simulink model "polyfitraspi"  (R2022a)
settings: Solver=VariableStepAuto  StartTime=0.0  StopTime=10.0  RelTol=1e-3
libraries: raspberrypiAVlib x2
settings Model: Creator=sanz  LastModifiedBy=sanz

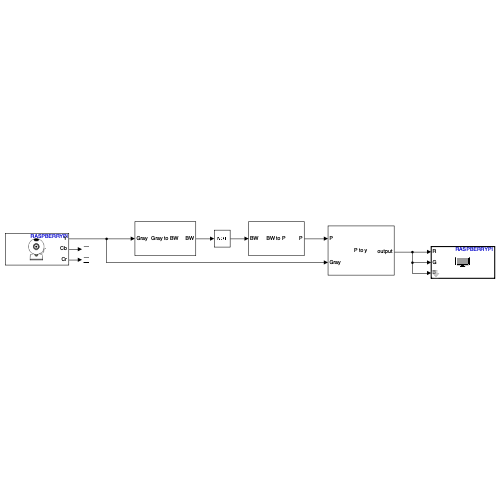
[thumbnail: Simulink's stored preview of the top-level diagram]
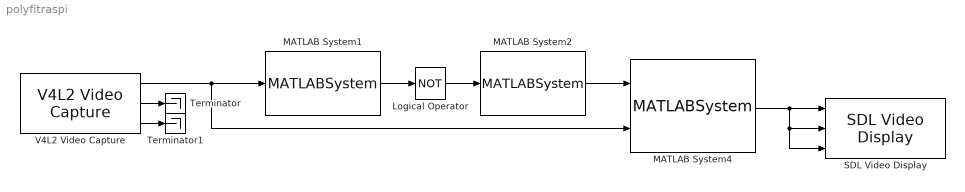
== system polyfitraspi ==
  Logical Operator : Logic  Operator=NOT  AllPortsSameDT=off  OutDataTypeStr=boolean
  MATLAB System1 : MATLABSystem  System=FrameBinarizeSystem  SimulateUsing=Code generation
      mask Type: FrameBinarizeSystem
      mask Display:
      | disp('Gray to BW');
      | port_label('input',1,'Gray');
      | port_label('output',1,'BW');
  MATLAB System2 : MATLABSystem  System=PolyfitSystem  Deg=4  SimulateUsing=Code generation
      mask Type: PolyfitSystem
      mask Display:
      | disp('BW to P');
      | port_label('input',1,'BW');
      | port_label('output',1,'P');
  MATLAB System4 : MATLABSystem  System=PolyvalSystem  SimulateUsing=Code generation
      mask Type: PolyvalSystem
      mask Display:
      | disp('P to y');
      | port_label('input',1,'P');
      | port_label('input',2,'Gray');
      | port_label('output',1,'output');
  SDL Video Display : raspberrypiAVlib/SDL Video Display  title=SDL Video Display  pixelFormat=RGB  pixelOrder=Planar  rowMajor=on  blockPlatform=Raspberry Pi
      settings: SourceProductBaseCode=SC_BEAGLEBONE_BLUE,EMBEDDEDLINUX,NVIDIA,RASPPIIO
  Terminator : Terminator
  Terminator1 : Terminator
  V4L2 Video Capture : raspberrypiAVlib/V4L2 Video Capture  DeviceName=/dev/video0  Resolution=320x240  CustomResolution=[ 320, 240 ]  PixelFormat=YCbCr 4:2:2  SampleTime=0.1  pixelOrder=planar  simOutput=Colorbars  imSizeSelection=320x240  imSize=[640, 480]  roi=[0, 0, 640, 480]  m_devName='/dev/video0'  blockPlatform=LINUX  HorizontalFlip=off  VerticalFlip=off  Brightness=0.5  Saturation=0.5  Contrast=0.5  Sharpness=0.5  CameraPan=0  CameraTilt=0  CameraZoom=0.5  EnableManualFocus=on  ManualFocus=0.5
      settings: SourceProductBaseCode=RASPPI
  wires:
  MATLAB System4/1 -> SDL Video Display/3, SDL Video Display/2, SDL Video Display/1
  MATLAB System1/1 -> Logical Operator/1
  MATLAB System2/1 -> MATLAB System4/1
  Logical Operator/1 -> MATLAB System2/1
  V4L2 Video Capture/1 -> MATLAB System1/1, MATLAB System4/2
  V4L2 Video Capture/3 -> Terminator1/1
  V4L2 Video Capture/2 -> Terminator/1
